simulink model "Fig522M5G50"  (R2014b)
settings: Solver=ode3  StartTime=0.0  StopTime=10.001  FixedStep=2e-7  RelTol=1e-3
libraries: commseqgen2 x4, commsink2 x2, commfilt2 x2, commanapbnd3 x2, commrandsrc2 x2, commchan3 x1
settings Model: Creator=Silage  LastModifiedBy=Silage

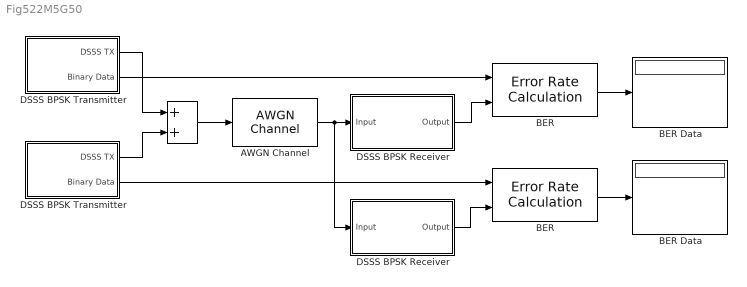
== system Fig522M5G50 ==
  " " : Sum
  " BER " : commsink2/Error Rate Calculation  N=2  st_delay=0  cp_mode=Entire frame  subframe=[]  PMode=Port  WsName=ErrorVec  RsMode2=off  stop=off  numErr=100  maxBits=1e6
  " BER Data " : Display
  AWGN Channel : commchan3/AWGN Channel  InputProcessing=Columns as channels (frame based)  seed=randseed  noiseMode="Signal to noise ratio  (Eb/No)"  EbNodB=80  EsNodB=10  SNRdB=0  bitsPerSym=1  Ps=12.5  Tsym=1e-3  variance=100000
  BER : commsink2/Error Rate Calculation  N=2  st_delay=0  cp_mode=Entire frame  subframe=[]  PMode=Port  WsName=ErrorVec  RsMode2=off  stop=off  numErr=100  maxBits=1e6
  BER Data : Display
  "DSSS BPSK Receiver  " : Subsystem
  "DSSS BPSK Transmitter " : Subsystem
  DSSS BPSK Receiver : Subsystem
  DSSS BPSK Transmitter : Subsystem
  wires:
  BER/1 -> BER Data/1
  " BER "/1 -> " BER Data "/1
  DSSS BPSK Receiver/1(Output) -> " BER "/2
  DSSS BPSK Transmitter/2("Binary Data ") -> " BER "/1
  "DSSS BPSK Transmitter "/2("Binary Data ") -> BER/1
  "DSSS BPSK Receiver  "/1(Output) -> BER/2
  "DSSS BPSK Transmitter "/1(DSSS TX) -> " "/2
  DSSS BPSK Transmitter/1(DSSS TX) -> " "/1
  AWGN Channel/1 -> "DSSS BPSK Receiver  "/1(Input), DSSS BPSK Receiver/1(Input)
  " "/1 -> AWGN Channel/1

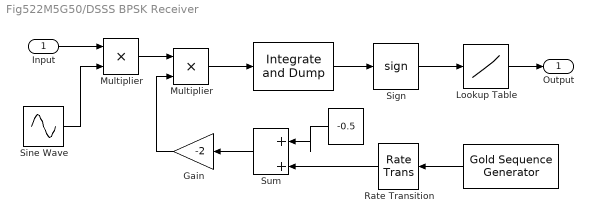
== system Fig522M5G50/DSSS BPSK Receiver   ==
  Input : Inport
  " " : Constant  Value=-0.5
  "   " : commseqgen2/Gold Sequence Generator  genPoly1=[1 0 0 1 0 1]  iniState1=[1 0 1 0 1]  genPoly2=[1 1 1 1 0 1]  iniState2=[1 1 1 0 0]  index=0  shift=0  outVarSiz=off  maxOutSizeMode=Dialog parameter  maxOutSize=[10 1]  ts=2e-5  frameBased=off  sampPerFrame=1  reset=off  outDataType=double
  "    " : commfilt2/Integrate and Dump  obssamples=5000  offsetsamples=0  nodump=off  roundingMode=Floor  overflowMode=off
  " Lookup Table" : Lookup_n-D  NumberOfTableDimensions=1  BreakpointsForDimension1=[-1, 0, 1]  BreakpointsForDimension3=[5, 7]  Table=[0, 0, 1]  InternalRulePriority=Speed  RndMeth=Simplest  InputSameDT=on
  Gain : Gain  Gain=-2
  "Multiplier " : Product
  "Multiplier " : Product
  "Rate Transition " : RateTransition  OutPortSampleTime=2e-7
  Sign : Signum
  Sine Wave : Sin  Amplitude=5  Frequency=200000*pi  Phase=pi/2  SampleTime=2e-7
  Sum : Sum  Inputs=|++
  Output : Outport
  wires:
  Sign/1 -> " Lookup Table"/1
  Input/1 -> "Multiplier "/1
  Sine Wave/1 -> "Multiplier "/2
  "    "/1 -> Sign/1
  Sum/1 -> Gain/1
  "Multiplier "/1 -> "    "/1
  "   "/1 -> "Rate Transition "/1
  "Multiplier "/1 -> "Multiplier "/1
  Gain/1 -> "Multiplier "/2
  "Rate Transition "/1 -> Sum/2
  " "/1 -> Sum/1
  " Lookup Table"/1 -> Output/1

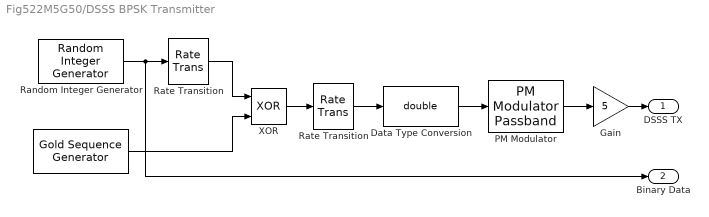
== system Fig522M5G50/DSSS BPSK Transmitter  ==
  " " : commseqgen2/Gold Sequence Generator  genPoly1=[1 0 0 1 0 1]  iniState1=[1 0 1 0 1]  genPoly2=[1 1 1 1 0 1]  iniState2=[1 1 1 0 0]  index=0  shift=0  outVarSiz=off  maxOutSizeMode=Dialog parameter  maxOutSize=[10 1]  ts=2e-5  frameBased=off  sampPerFrame=1  reset=off  outDataType=double
  Data Type Conversion : DataTypeConversion  OutDataTypeStr=double
  Gain : Gain  Gain=5
  PM Modulator : commanapbnd3/PM Modulator Passband  Fc=100000  Ph=pi  Kc=pi
  Random Integer Generator : commrandsrc2/Random Integer Generator  mul=2  seed=49  Ts=1e-3  frameBased=off  sampPerFrame=50  orient=on  outDataType=double
  "Rate Transition " : RateTransition  OutPortSampleTime=2e-7
  Rate Transition : RateTransition  OutPortSampleTime=2e-5
  XOR : Logic  Operator=XOR  IconShape=distinctive  AllPortsSameDT=off  OutDataTypeStr=boolean
  DSSS TX : Outport
  "Binary Data " : Outport  Port=2
  wires:
  " "/1 -> XOR/2
  Random Integer Generator/1 -> Rate Transition/1, "Binary Data "/1
  Rate Transition/1 -> XOR/1
  Data Type Conversion/1 -> PM Modulator/1
  XOR/1 -> "Rate Transition "/1
  "Rate Transition "/1 -> Data Type Conversion/1
  PM Modulator/1 -> Gain/1
  Gain/1 -> DSSS TX/1

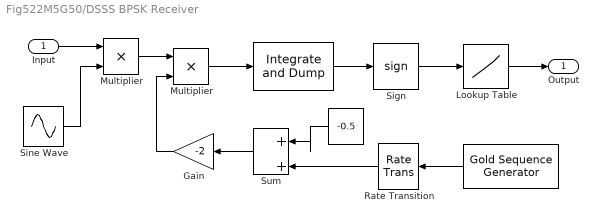
== system Fig522M5G50/DSSS BPSK Receiver ==
  Input : Inport
  " " : Constant  Value=-0.5
  "   " : commseqgen2/Gold Sequence Generator  genPoly1=[1 0 0 1 0 1]  iniState1=[1 1 1 0 1]  genPoly2=[1 1 1 1 0 1]  iniState2=[1 0 0 0 1]  index=0  shift=0  outVarSiz=off  maxOutSizeMode=Dialog parameter  maxOutSize=[10 1]  ts=2e-5  frameBased=off  sampPerFrame=1  reset=off  outDataType=double
  "    " : commfilt2/Integrate and Dump  obssamples=5000  offsetsamples=0  nodump=off  roundingMode=Floor  overflowMode=off
  " Lookup Table" : Lookup_n-D  NumberOfTableDimensions=1  BreakpointsForDimension1=[-1, 0, 1]  BreakpointsForDimension3=[5, 7]  Table=[0, 0, 1]  InternalRulePriority=Speed  RndMeth=Simplest  InputSameDT=on
  Gain : Gain  Gain=-2
  "Multiplier " : Product
  "Multiplier " : Product
  "Rate Transition " : RateTransition  OutPortSampleTime=2e-7
  Sign : Signum
  Sine Wave : Sin  Amplitude=5  Frequency=200000*pi  Phase=pi/2  SampleTime=2e-7
  Sum : Sum  Inputs=|++
  Output : Outport
  wires:
  Sign/1 -> " Lookup Table"/1
  Input/1 -> "Multiplier "/1
  Sine Wave/1 -> "Multiplier "/2
  "    "/1 -> Sign/1
  Sum/1 -> Gain/1
  "Multiplier "/1 -> "    "/1
  "   "/1 -> "Rate Transition "/1
  "Multiplier "/1 -> "Multiplier "/1
  Gain/1 -> "Multiplier "/2
  "Rate Transition "/1 -> Sum/2
  " "/1 -> Sum/1
  " Lookup Table"/1 -> Output/1

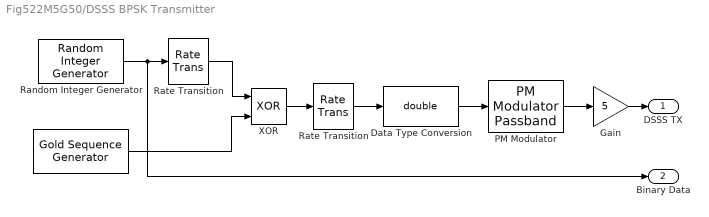
== system Fig522M5G50/DSSS BPSK Transmitter ==
  " " : commseqgen2/Gold Sequence Generator  genPoly1=[1 0 0 1 0 1]  iniState1=[1 1 1 0 1]  genPoly2=[1 1 1 1 0 1]  iniState2=[1 0 0 0 1]  index=0  shift=0  outVarSiz=off  maxOutSizeMode=Dialog parameter  maxOutSize=[10 1]  ts=2e-5  frameBased=off  sampPerFrame=1  reset=off  outDataType=double
  Data Type Conversion : DataTypeConversion  OutDataTypeStr=double
  Gain : Gain  Gain=5
  PM Modulator : commanapbnd3/PM Modulator Passband  Fc=100000  Ph=pi  Kc=pi
  Random Integer Generator : commrandsrc2/Random Integer Generator  mul=2  seed=37  Ts=1e-3  frameBased=off  sampPerFrame=50  orient=on  outDataType=double
  "Rate Transition " : RateTransition  OutPortSampleTime=2e-7
  Rate Transition : RateTransition  OutPortSampleTime=2e-5
  XOR : Logic  Operator=XOR  IconShape=distinctive  AllPortsSameDT=off  OutDataTypeStr=boolean
  DSSS TX : Outport
  "Binary Data " : Outport  Port=2
  wires:
  Rate Transition/1 -> XOR/1
  Data Type Conversion/1 -> PM Modulator/1
  XOR/1 -> "Rate Transition "/1
  "Rate Transition "/1 -> Data Type Conversion/1
  PM Modulator/1 -> Gain/1
  Gain/1 -> DSSS TX/1
  Random Integer Generator/1 -> "Binary Data "/1, Rate Transition/1
  " "/1 -> XOR/2
